simulink model "UNIFIER_dyn3DOF"  (R2023b)
settings: Solver=VariableStepAuto  StartTime=0.0  StopTime=0  RelTol=1e-3
InitFcn:
  | UNIFIER_LOAD
values from neighbouring files (symbols this model uses):
  b = 20.11467    [UNIFIER_LOAD.m]    (also in UNIFIER_LOAD.mat; UNIFIER_LOAD_ROM.m; UNIFIER_LOAD_ROM.mat)
  c = 1.43676    [UNIFIER_LOAD.m]    (also in UNIFIER_LOAD.mat; UNIFIER_LOAD_ROM.m; UNIFIER_LOAD_ROM.mat)
  dp_DEP =     [UNIFIER_LOAD.mat]    (also in UNIFIER_LOAD_ROM.mat)
  dp_FUSE_FIN =     [UNIFIER_LOAD.mat]
  dp_HTU =     [UNIFIER_LOAD.mat]    (also in UNIFIER_LOAD_ROM.mat)
  dp_VTAIL =     [UNIFIER_LOAD.mat]
  dp_VTAIL_INDUCED =     [UNIFIER_LOAD.mat]
  dp_WING_root =     [UNIFIER_LOAD.mat]
  dp_WING_tip =     [UNIFIER_LOAD.mat]
  I = [23600,     -0,  -1740 ... (first row only)    [UNIFIER_LOAD.m]    (also in UNIFIER_LOAD.mat = [23600  0  -1740; 0  89800  0; -1740  0  102000]; UNIFIER_LOAD_ROM.m = [23600,     -0,   -1740; UNIFIER_LOAD_ROM.mat = [23600  0  -1740; 0  89800  0; -1740  0  102000])
  m = 7057    [UNIFIER_LOAD.m]    (also in UNIFIER_LOAD.mat; UNIFIER_LOAD_ROM.m; UNIFIER_LOAD_ROM.mat)
  S = 29.98388    [UNIFIER_LOAD.m]    (also in UNIFIER_LOAD.mat; UNIFIER_LOAD_ROM.m; UNIFIER_LOAD_ROM.mat)
  vtail_nodes = [dp_VTAIL.Xs_LE;     dp_VTAIL.Ys_LE;     dp_VTAIL.Zs_LE]    [UNIFIER_LOAD.m]    (also in UNIFIER_LOAD.mat = [-16.4894695282 -2.83441376686 -2.73765826225 -16.1370849609)
  wing_nodes = [fliplr(dp_WING_tip.LE_Xs),fliplr(dp_WING_root.LE_Xs),dp_WING_root.LE_Xs,dp_WING_tip.LE_Xs;     fliplr(-dp_WING_tip.LE_Ys),fliplr(-dp_WING_root.LE_Ys),dp_WING_root.LE_Ys,dp_WING_tip.LE_Ys;     fliplr(dp_WING_tip.LE_Zs),fliplr(dp_WING_root.LE_Zs),dp_WING_root.LE_Zs,dp_WING_tip.LE_Zs]    [UNIFIER_LOAD.m]    (also in UNIFIER_LOAD.mat = [-7.70795631409 -9.67500019073 -0.98178178072 -7.66801691055)
  xyz_cg = [-8.09,0,-0.2]    [UNIFIER_LOAD.m]    (also in UNIFIER_LOAD.mat = [-8.09 0 -0.2]; UNIFIER_LOAD_ROM.m; UNIFIER_LOAD_ROM.mat = [-8.09 0 -0.2])
  xyz_DEP = [ -6.9629998	-6.9210000	-6.8660002	-6.8099999	-6.7540002	-6.6999998	-6.6999998	-6.7540002	-6.8099999	-6.8660002	-6.9210000	-6.9629998 ... (first row only)    [UNIFIER_LOAD.m]    (also in UNIFIER_LOAD.mat = [-6.9629998 -10.05 -0.90899998 -6.921 -8.4499998 -0.792 -6.8; UNIFIER_LOAD_ROM.m; UNIFIER_LOAD_ROM.mat = [-6.9629998 -10.05 -0.90899998 -6.921 -8.4499998 -0.792 -6.8)
undefined symbols (not defined in the file or in its folder): OBM, unifier_obm
libraries: sharedutil x7, aerolibtransform2 x4, sharedtransform x2, aerolibatmos2 x1, matrix_library x1, shared6dofsys x1, shared6dof x1, simulink x1
(part 3 of 3)

== system UNIFIER_dyn3DOF/UNIFIER OBM1/Aero/WingForces/Right/Subsystem/CrossProduct ==
  r : Inport  Partition=on  PartitionDimension=2  PartitionWidth=1  PartitionOffset=0
  F : Inport  Port=2  Partition=on  PartitionDimension=2  PartitionWidth=1  PartitionOffset=0
  3x3 Cross Product : sharedutil/3x3 Cross Product  aMode=aMode
  CG : Constant  Value=xyz_cg
  Cast : DataTypeConversion  OutDataTypeStr=single  SaturateOnIntegerOverflow=off  RndMeth=Floor
  For Each : ForEach  DisableCoverage=on  SpecifiedNumIters=7
  Minus : Sum  Inputs=+-
  M : Outport  ConcatenationDimension=2
  wires:
  Cast/1 -> Minus/2
  Minus/1 -> 3x3 Cross Product/1
  CG/1 -> Cast/1
  3x3 Cross Product/1 -> M/1
  r/1 -> Minus/1
  F/1 -> 3x3 Cross Product/2

== system UNIFIER_dyn3DOF/UNIFIER OBM1/Aero/WingForces/Right/Subsystem/w2b ==
  alpha : Inport  OutDataTypeStr=single  Partition=on  PartitionDimension=1  PartitionWidth=1  PartitionOffset=0
  Fw : Inport  Port=2  Partition=on  PartitionDimension=2  PartitionWidth=1  PartitionOffset=0
  Cast To Double : DataTypeConversion  OutDataTypeStr=double  SaturateOnIntegerOverflow=off  RndMeth=Floor
  Cast To Single : DataTypeConversion  OutDataTypeStr=single  SaturateOnIntegerOverflow=off  RndMeth=Floor
  Constant : Constant  Value=0  OutDataTypeStr=single
  Demux : Demux  Outputs=3
  Direction Cosine Matrix Body to Wind : aerolibtransform2/Direction Cosine Matrix Body to Wind
  Display : Display
  Display1 : Display
  For Each : ForEach  DisableCoverage=on  SpecifiedNumIters=7
  Matrix Multiply : Product  Multiplication=Matrix(*)
  Mux : Mux  Inputs=3
  Mux1 : Mux  Inputs=2
  Transpose : Math  Operator=transpose
  Unary Minus : UnaryMinus
  Unary Minus1 : UnaryMinus
  Fb : Outport  ConcatenationDimension=2
  wires:
  Cast To Double/1 -> Direction Cosine Matrix Body to Wind/1
  Cast To Single/1 -> Matrix Multiply/1
  Constant/1 -> Mux1/2
  Mux1/1 -> Cast To Double/1
  Transpose/1 -> Cast To Single/1
  Direction Cosine Matrix Body to Wind/1 -> Transpose/1
  Demux/3 -> Unary Minus1/1
  Unary Minus1/1 -> Mux/3
  Demux/2 -> Mux/2
  Unary Minus/1 -> Mux/1
  Demux/1 -> Unary Minus/1
  Mux/1 -> Matrix Multiply/2
  Matrix Multiply/1 -> Fb/1
  alpha/1 -> Mux1/1, Display/1
  Fw/1 -> Demux/1, Display1/1

== system UNIFIER_dyn3DOF/UNIFIER OBM1/Aero/WingForces/Right/WingRootForces/WingRootPreLookup ==
  flap_defl : Inport
  alpha : Inport  Port=2
  V_node : Inport  Port=3
  DEP_J : Inport  Port=4
  Constant8 : Constant  Value=0:4
  Prelookup : PreLookup  BreakpointsData=dp_WING_root.flap_defl  IndexSearchMethod=Linear search  BeginIndexSearchUsingPreviousIndexResult=on  UseLastBreakpoint=on
  Prelookup1 : PreLookup  BreakpointsData=dp_WING_root.alphas  IndexSearchMethod=Linear search  BeginIndexSearchUsingPreviousIndexResult=on  UseLastBreakpoint=on
  Prelookup2 : PreLookup  BreakpointsData=dp_WING_root.V  IndexSearchMethod=Linear search  BeginIndexSearchUsingPreviousIndexResult=on  UseLastBreakpoint=on
  Prelookup3 : PreLookup  BreakpointsData=dp_WING_root.DEP_J  IndexSearchMethod=Linear search  BeginIndexSearchUsingPreviousIndexResult=on  UseLastBreakpoint=on
  Out1 : Outport
  Out2 : Outport  Port=2
  Out3 : Outport  Port=3
  Out4 : Outport  Port=4
  Out6 : Outport  Port=5
  Out7 : Outport  Port=6
  Out8 : Outport  Port=7
  Out9 : Outport  Port=8
  Out5 : Outport  Port=9
  wires:
  Prelookup3/2 -> Out9/1
  Prelookup3/1 -> Out8/1
  Prelookup2/2 -> Out7/1
  Prelookup2/1 -> Out6/1
  DEP_J/1 -> Prelookup3/1
  V_node/1 -> Prelookup2/1
  flap_defl/1 -> Prelookup/1
  Prelookup1/1 -> Out3/1
  alpha/1 -> Prelookup1/1
  Prelookup/2 -> Out2/1
  Prelookup1/2 -> Out4/1
  Constant8/1 -> Out5/1
  Prelookup/1 -> Out1/1

== system UNIFIER_dyn3DOF/UNIFIER OBM1/Aero/WingForces/Right/WingTipForces/WingRootPreLookup ==
  ail_defl : Inport
  alpha : Inport  Port=2
  V_node : Inport  Port=3
  DEP_J : Inport  Port=4
  Constant8 : Constant  Value=0:1
  Prelookup : PreLookup  BreakpointsData=dp_WING_tip.ail_defl  IndexSearchMethod=Linear search  BeginIndexSearchUsingPreviousIndexResult=on  UseLastBreakpoint=on
  Prelookup1 : PreLookup  BreakpointsData=dp_WING_tip.alphas  IndexSearchMethod=Linear search  BeginIndexSearchUsingPreviousIndexResult=on  UseLastBreakpoint=on
  Prelookup2 : PreLookup  BreakpointsData=dp_WING_tip.V  IndexSearchMethod=Linear search  BeginIndexSearchUsingPreviousIndexResult=on  UseLastBreakpoint=on
  Prelookup3 : PreLookup  BreakpointsData=dp_WING_tip.DEP_J  IndexSearchMethod=Linear search  BeginIndexSearchUsingPreviousIndexResult=on  UseLastBreakpoint=on
  Out1 : Outport
  Out2 : Outport  Port=2
  Out3 : Outport  Port=3
  Out4 : Outport  Port=4
  Out6 : Outport  Port=5
  Out7 : Outport  Port=6
  Out8 : Outport  Port=7
  Out9 : Outport  Port=8
  Out5 : Outport  Port=9
  wires:
  Prelookup3/2 -> Out9/1
  Prelookup3/1 -> Out8/1
  Prelookup2/2 -> Out7/1
  Prelookup2/1 -> Out6/1
  DEP_J/1 -> Prelookup3/1
  V_node/1 -> Prelookup2/1
  ail_defl/1 -> Prelookup/1
  Prelookup1/1 -> Out3/1
  alpha/1 -> Prelookup1/1
  Prelookup/2 -> Out2/1
  Prelookup1/2 -> Out4/1
  Constant8/1 -> Out5/1
  Prelookup/1 -> Out1/1
